simulink model "Square"  (R2012b)
settings: Solver=ode1  StartTime=0.0  StopTime=inf  FixedStep=0.002  RelTol=1e-3
undefined symbols (not defined in the file): qc_get_step_size
libraries: simulink x33, simulink_extras x8, quarc_library x2
settings Model: ExtModeTrigDuration=5000  Creator=user  LastModifiedBy=user
settings SolverCC: PositivePriorityOrder=on
settings RTWCC: SystemTargetFile=quarc_win64.tlc  TemplateMakefile=quarc_default_tmf  Description=QUARC Win64 Target  ProcessScript=quarc_win64_make_rtw_hook
settings STFCustomTargetCC: TargetPreCompLibLocation=C:\PROGRA~3\QUARC\lib\2012b\win64\release  CodeReplacementLibrary=ANSI_C  GeneratePreprocessorConditionals=Disable all  CombineOutputUpdateFcns=on  GRTInterface=off  SystemTargetFile=quarc_win64.tlc
settings GRTTargetCC: TargetPreCompLibLocation=C:\PROGRA~3\QUARC\lib\2012b\win64\release  ParMdlRefBuildCompliant=off  CompOptLevelCompliant=off  ConcurrentExecutionCompliant=off  MatFileLogging=off  ExtMode=on  ExtModeMexFile=quarc_comm

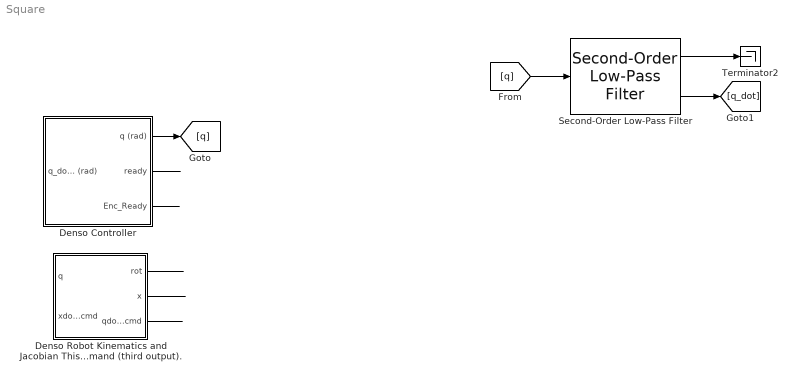
== system Square ==
  Denso Controller : Subsystem
  Denso Robot Kinematics and Jacobian This block takes the joint values of the robot as the first input and calculates the rotational matrix and position of the robot end-effector in the global frame (first two outputs). It also takes the speed command in the global frame (second input) and converts it to joint speed command (third output). : Subsystem
  Second-Order Low-Pass Filter : quarc_library/Continuous/Second-Order Low-Pass Filter  params_source=Internal (dialog parameters)  input_width=1  input_zeta=1  input_init=0
  Terminator2 : Terminator
  wires:
  [q] -> Second-Order Low-Pass Filter/1
  Denso Controller/1(q (rad)) -> [q]
  Second-Order Low-Pass Filter/1 -> Terminator2/1
  Second-Order Low-Pass Filter/2 -> [q_dot]
  Denso Robot Kinematics and Jacobian This block takes the joint values of the robot as the first input and calculates the rotational matrix and position of the robot end-effector in the global frame (first two outputs). It also takes the speed command in the global frame (second input) and converts it to joint speed command (third output)./1(rot) -> ?
  Denso Robot Kinematics and Jacobian This block takes the joint values of the robot as the first input and calculates the rotational matrix and position of the robot end-effector in the global frame (first two outputs). It also takes the speed command in the global frame (second input) and converts it to joint speed command (third output)./2(x) -> ?
  Denso Controller/2(ready) -> ?
  Denso Controller/3(Enc_Ready) -> ?
  ? -> Denso Controller/1(q_dot_cmd (rad))
  Denso Robot Kinematics and Jacobian This block takes the joint values of the robot as the first input and calculates the rotational matrix and position of the robot end-effector in the global frame (first two outputs). It also takes the speed command in the global frame (second input) and converts it to joint speed command (third output)./3(qdot_cmd) -> ?

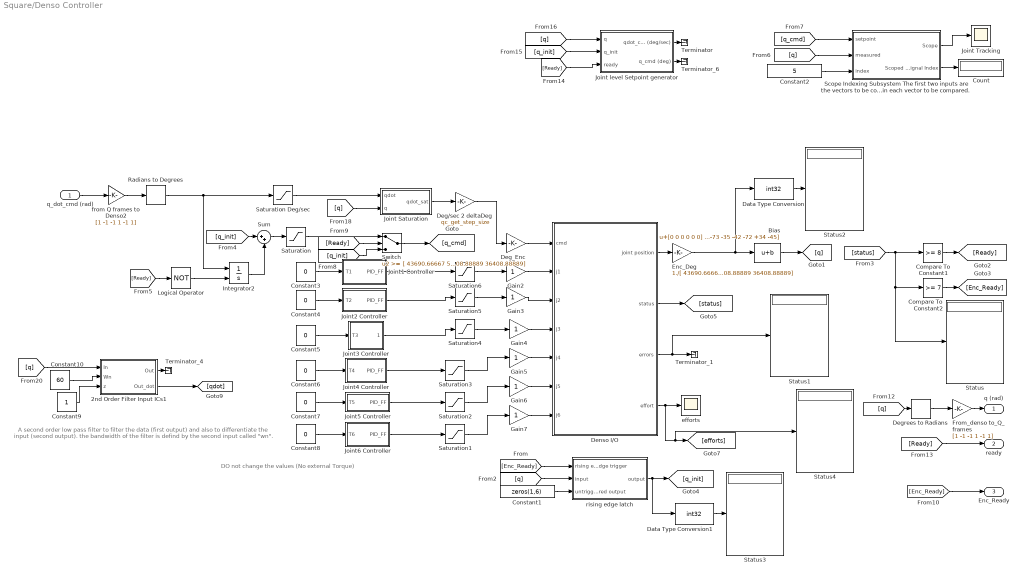
== system Square/Denso Controller ==
  note: DO not change the values (No external Torque)
  note: A second order low pass filter to filter the data (first output) and also to differentiate
      |  the input (second output). the bandwidth of the filter is defind by the second input called "wn".
  q_dot_cmd (rad) : Inport
  2nd Order Filter Input ICs1 : Subsystem
  Bias : Bias  Bias=[0 0 0 0 0 0] %0*[-146 -102 -137+90 -155 85+90 -370]%[-73 -35 -42 -72 +34 -45]
  Compare To Constant1 : simulink/Logic and Bit Operations/Compare To Constant  relop=>=  const=8  OutDataTypeStr=uint8  ZeroCross=off
  Compare To Constant2 : simulink/Logic and Bit Operations/Compare To Constant  relop=>=  const=7  OutDataTypeStr=uint8  ZeroCross=off
  Constant1 : Constant  Value=zeros(1,6)
  Constant10 : Constant  Value=60
  Constant2 : Constant  Value=5
  Constant{3..8} (6 alike) : Constant  Value=0
  Constant9 : Constant
  Count : Display
      settings: Decimation=100
  Data Type Conversion : DataTypeConversion  OutDataTypeStr=int32
  Data Type Conversion1 : DataTypeConversion  OutDataTypeStr=int32
  Deg/sec 2 deltaDeg : Gain  Gain=qc_get_step_size
  Deg_Enc : Gain  Gain=[ 43690.66667 58254.22222 43690.66667 36408.88889 36408.88889 36408.88889]
  Degrees to Radians : simulink_extras/Transformations/Degrees to Radians
  Denso I/O : Subsystem
  Enc_Deg : Gain  Gain=1./[ 43690.66667 58254.22222 43690.66667 36408.88889 36408.88889 36408.88889]
  From_denso to_Q_frames : Gain  Gain=[1 -1 -1 1 -1 1]
  Gain{2..7} (6 alike) : Gain
  Integrator2 : Integrator  ExternalReset=level
  Joint Saturation : Subsystem
  Joint Tracking : Scope
      settings: TimeRange=2  YMin=93  YMax=100.5
  Joint level Setpoint generator : Subsystem
  Joint1 Controller : Subsystem
  Joint2 Controller : Subsystem
  Joint3 Controller : Subsystem
  Joint4 Controller : Subsystem
  Joint5 Controller : Subsystem
  Joint6 Controller : Subsystem
  Logical Operator : Logic  Operator=NOT  AllPortsSameDT=off  OutDataTypeStr=boolean
  Radians to Degrees : simulink_extras/Transformations/Radians to Degrees
  Saturation : Saturate  UpperLimit=[160 65 162 162 100 365]  LowerLimit=-[160 122 20 162 100 365]
  Saturation Deg/sec : Saturate  UpperLimit="1e3*[1.1444    0.8583    1.1444    1.3733    1.3733    1.3733]"  LowerLimit="-1e3*[1.1444    0.8583    1.1444    1.3733    1.3733    1.3733]"
  Saturation{1..6} (6 alike) : Saturate  UpperLimit=3.7  LowerLimit=-3.7
  Scope Indexing Subsystem The first two inputs are the vectors to be compared. The third input is an index to define the elements in each vector to be compared. : Subsystem
  Status{,1..4} (5 alike) : Display
      settings: Decimation=100
  Sum : Sum  Inputs=|++
  Switch : Switch  Threshold=1
  Terminator : Terminator
  Terminator_1 : Terminator
  Terminator_4 : Terminator
  Terminator_6 : Terminator
  efforts : Scope
      settings: TimeRange=2  YMin=-4.5  YMax=0.5  SaveName=ScopeData3
  from Q frames to Denso2 : Gain  Gain=[1 -1 -1 1 -1 1]
  rising edge latch : Subsystem
  q (rad) : Outport
  ready : Outport  Port=2
  Enc_Ready : Outport  Port=3
  wires:
  Denso I/O/1(joint position) -> Enc_Deg/1
  Enc_Deg/1 -> Data Type Conversion/1, Bias/1
  Gain2/1 -> Denso I/O/2(j1)
  Gain3/1 -> Denso I/O/3(j2)
  Gain4/1 -> Denso I/O/4(j3)
  Gain5/1 -> Denso I/O/5(j4)
  Gain6/1 -> Denso I/O/6(j5)
  Gain7/1 -> Denso I/O/7(j6)
  Joint2 Controller/1(PID_FF) -> Saturation5/1
  Joint3 Controller/1(PID_FF) -> Saturation4/1
  Joint1 Controller/1(PID_FF) -> Saturation6/1
  [Enc_Ready] -> rising edge latch/1(rising edge trigger)
  Compare To Constant1/1 -> [Ready]
  [q] -> rising edge latch/2(input)
  rising edge latch/1(output) -> [q_init], Data Type Conversion1/1
  Constant1/1 -> rising edge latch/3(untriggered output)
  Denso I/O/4(effort) -> efforts/1, [efforts], Status4/1
  Scope Indexing Subsystem The first two inputs are the vectors to be compared. The third input is an index to define the elements in each vector to be compared./2(Scoped Signal Index) -> Count/1
  Constant2/1 -> Scope Indexing Subsystem The first two inputs are the vectors to be compared. The third input is an index to define the elements in each vector to be compared./3(index)
  Compare To Constant2/1 -> [Enc_Ready]
  Denso I/O/2(status) -> [status]
  [status] -> Compare To Constant1/1, Compare To Constant2/1, Status/1
  [q_cmd] -> Scope Indexing Subsystem The first two inputs are the vectors to be compared. The third input is an index to define the elements in each vector to be compared./1(setpoint)
  [q] -> Scope Indexing Subsystem The first two inputs are the vectors to be compared. The third input is an index to define the elements in each vector to be compared./2(measured)
  [Ready] -> Logical Operator/1
  Logical Operator/1 -> Integrator2/2
  q_dot_cmd (rad)/1 -> from Q frames to Denso2/1
  [q] -> Degrees to Radians/1
  [Ready] -> ready/1
  [Enc_Ready] -> Enc_Ready/1
  Denso I/O/3(errors) -> Terminator_1/1, Status1/1
  Degrees to Radians/1 -> From_denso to_Q_frames/1
  Deg/sec 2 deltaDeg/1 -> Deg_Enc/1
  From_denso to_Q_frames/1 -> q (rad)/1
  [q] -> 2nd Order Filter Input ICs1/1(In)
  Constant9/1 -> 2nd Order Filter Input ICs1/3(z)
  Constant10/1 -> 2nd Order Filter Input ICs1/2(Wn)
  2nd Order Filter Input ICs1/2(Out_dot) -> [qdot]
  Joint4 Controller/1(PID_FF) -> Saturation3/1
  Joint5 Controller/1(PID_FF) -> Saturation2/1
  Joint6 Controller/1(PID_FF) -> Saturation1/1
  2nd Order Filter Input ICs1/1(Out) -> Terminator_4/1
  [q] -> Joint level Setpoint generator/1(q)
  [q_init] -> Joint level Setpoint generator/2(q_init)
  [Ready] -> Joint level Setpoint generator/3(ready)
  Joint level Setpoint generator/2(q_cmd (deg)) -> Terminator_6/1
  Saturation Deg/sec/1 -> Joint Saturation/1(qdot)
  [q] -> Joint Saturation/2(q)
  from Q frames to Denso2/1 -> Radians to Degrees/1
  Scope Indexing Subsystem The first two inputs are the vectors to be compared. The third input is an index to define the elements in each vector to be compared./1(Scope) -> Joint Tracking/1
  Data Type Conversion/1 -> Status2/1
  Data Type Conversion1/1 -> Status3/1
  Joint Saturation/1(qdot_sat) -> Deg/sec 2 deltaDeg/1
  Bias/1 -> [q]
  [Ready] -> Switch/2
  Sum/1 -> Saturation/1
  Switch/1 -> [q_cmd]
  [q_init] -> Switch/3
  [q_init] -> Sum/1
  Integrator2/1 -> Sum/2
  Saturation/1 -> Switch/1
  Radians to Degrees/1 -> Integrator2/1, Saturation Deg/sec/1
  Deg_Enc/1 -> Denso I/O/1(cmd)
  Constant3/1 -> Joint1 Controller/1(T1)
  Constant4/1 -> Joint2 Controller/1(T2)
  Constant5/1 -> Joint3 Controller/1(T3)
  Constant6/1 -> Joint4 Controller/1(T4)
  Constant7/1 -> Joint5 Controller/1(T5)
  Saturation1/1 -> Gain7/1
  Saturation2/1 -> Gain6/1
  Saturation3/1 -> Gain5/1
  Saturation4/1 -> Gain4/1
  Saturation5/1 -> Gain3/1
  Saturation6/1 -> Gain2/1
  Constant8/1 -> Joint6 Controller/1(T6)
  Joint level Setpoint generator/1(qdot_cmd (deg/sec)) -> Terminator/1

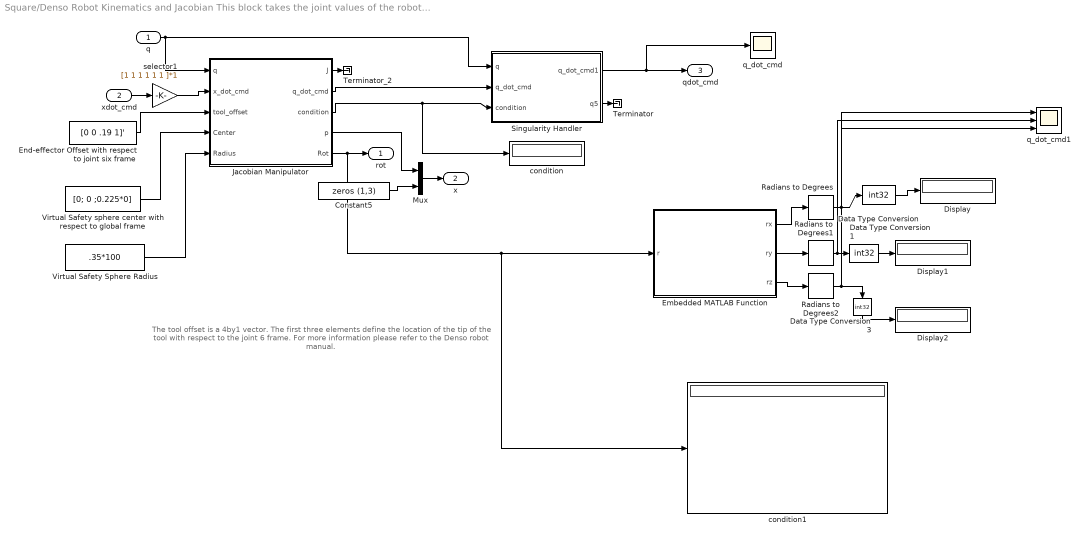
== system Square/Denso Robot Kinematics and Jacobian This block takes the joint values of the robot as the first input and calculates the rotational matrix and position of the robot end-effector in the global frame (first two outputs). It also takes the speed command in the global frame (second input) and converts it to joint speed command (third output). ==
  note: The tool offset is a 4by1 vector. The first three elements define
      | the location of the tip of the tool with respect to the joint 6 frame.
      | For more information please refer to the Denso robot manual.
  q : Inport
  xdot_cmd : Inport  Port=2
  Constant5 : Constant  Value=zeros (1,3)
  Data Type Conversion : DataTypeConversion  OutDataTypeStr=int32
  Data Type Conversion1 : DataTypeConversion  OutDataTypeStr=int32
  Data Type Conversion3 : DataTypeConversion  OutDataTypeStr=int32
  Display : Display
      settings: Decimation=100
  Display1 : Display
      settings: Decimation=100
  Display2 : Display
      settings: Decimation=100
  Embedded MATLAB Function : MATLAB Function  TreatAsAtomicUnit=on
  End-effector Offset with respect to joint six frame : Constant  Value=[0 0 .19 1]'
  Jacobian Manipulator : Subsystem
  Mux : Mux  Inputs=2
  Radians to Degrees : simulink_extras/Transformations/Radians to Degrees
  Radians to Degrees1 : simulink_extras/Transformations/Radians to Degrees
  Radians to Degrees2 : simulink_extras/Transformations/Radians to Degrees
  Singularity Handler : Subsystem
  Terminator : Terminator
  Terminator_2 : Terminator
  Virtual Safety Sphere Radius : Constant  Value=.35*100
  Virtual Safety sphere center with respect to global frame : Constant  Value=[0; 0 ;0.225*0]
  condition : Display
      settings: Decimation=100
  condition1 : Display
      settings: Decimation=100
  q_dot_cmd : Scope
      settings: TimeRange=2  YMin=-2.75e-005  YMax=2.75e-005  SaveName=ScopeData19
  q_dot_cmd1 : Scope  NumInputPorts=3
      settings: TimeRange=2  YMin=-2.75e-005~-5~-5  YMax=2.75e-005~5~5  SaveName=ScopeData5
  selector1 : Gain  Gain=[1 1 1 1 1 1 ]*1
  rot : Outport
  x : Outport  Port=2
  qdot_cmd : Outport  Port=3
  wires:
  Jacobian Manipulator/1(J) -> Terminator_2/1
  Constant5/1 -> Mux/2
  selector1/1 -> Jacobian Manipulator/2(x_dot_cmd)
  Jacobian Manipulator/3(condition) -> Singularity Handler/3(condition), condition/1
  Jacobian Manipulator/4(p) -> Mux/1
  Singularity Handler/1(q_dot_cmd1) -> q_dot_cmd/1, qdot_cmd/1
  End-effector Offset with respect to joint six frame/1 -> Jacobian Manipulator/3(tool_offset)
  Jacobian Manipulator/2(q_dot_cmd) -> Singularity Handler/2(q_dot_cmd)
  q/1 -> Jacobian Manipulator/1(q), Singularity Handler/1(q)
  xdot_cmd/1 -> selector1/1
  Jacobian Manipulator/5(Rot) -> rot/1, Embedded MATLAB Function/1(r), condition1/1
  Mux/1 -> x/1
  Virtual Safety sphere center with respect to global frame/1 -> Jacobian Manipulator/4(Center)
  Virtual Safety Sphere Radius/1 -> Jacobian Manipulator/5(Radius)
  Embedded MATLAB Function/1(rx) -> Radians to Degrees/1
  Embedded MATLAB Function/2(ry) -> Radians to Degrees1/1
  Embedded MATLAB Function/3(rz) -> Radians to Degrees2/1
  Radians to Degrees/1 -> Data Type Conversion/1, q_dot_cmd1/1
  Radians to Degrees1/1 -> Data Type Conversion1/1, q_dot_cmd1/2
  Radians to Degrees2/1 -> Data Type Conversion3/1, q_dot_cmd1/3
  Data Type Conversion/1 -> Display/1
  Data Type Conversion1/1 -> Display1/1
  Data Type Conversion3/1 -> Display2/1
  Singularity Handler/2(q5) -> Terminator/1

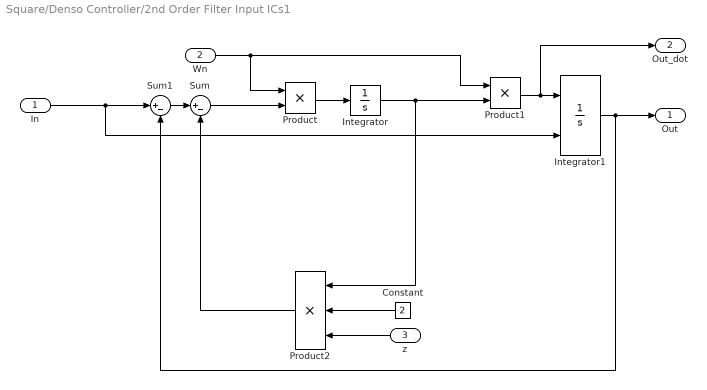
== system Square/Denso Controller/2nd Order Filter Input ICs1 ==
  In : Inport
  Wn : Inport  Port=2
  z : Inport  Port=3
  Constant : Constant  Value=2
  Integrator : Integrator
  Integrator1 : Integrator  InitialConditionSource=external
  Product : Product  RndMeth=Zero
  Product1 : Product  RndMeth=Zero
  Product2 : Product  Inputs=3  RndMeth=Zero
  Sum : Sum  Inputs=|+-
  Sum1 : Sum  Inputs=|+-
  Out : Outport
  Out_dot : Outport  Port=2
  wires:
  Constant/1 -> Product2/2
  z/1 -> Product2/3
  Product2/1 -> Sum/2
  In/1 -> Integrator1/2, Sum1/1
  Sum1/1 -> Sum/1
  Integrator1/1 -> Out/1, Sum1/2
  Integrator/1 -> Product2/1, Product1/2
  Product1/1 -> Out_dot/1, Integrator1/1
  Wn/1 -> Product1/1, Product/1
  Sum/1 -> Product/2
  Product/1 -> Integrator/1

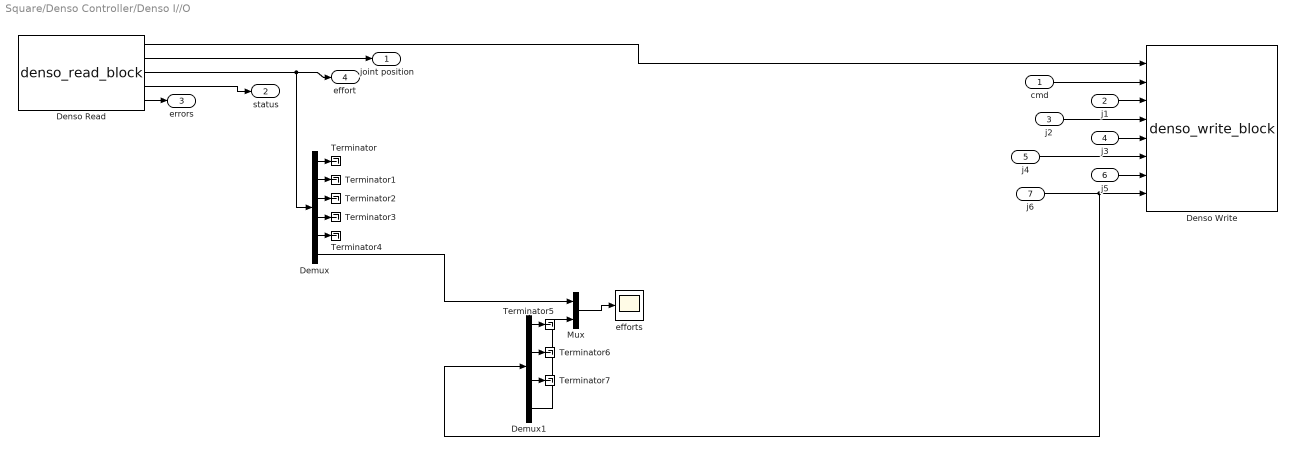
== system Square/Denso Controller/Denso I//O ==
  cmd : Inport
  j1 : Inport  Port=2
  j2 : Inport  Port=3
  j3 : Inport  Port=4
  j4 : Inport  Port=5
  j5 : Inport  Port=6
  j6 : Inport  Port=7
  Demux : Demux  Outputs=6
  Demux1 : Demux
  Denso Read : S-Function  FunctionName=denso_read_block  Parameters=uri  EnableBusSupport=off  mask(Denso Read){uri=udp://192.168.0.1:1000}
      mask help: Initializes a connection to the Denso robot controller and reads the robot joint positions and state.
      mask init:
      | commands = { ...
      |     'port_label(''output'', 1, ''denso'');', ...
      |     'port_label(''output'', 2, ''position'');', ...
      |     'port_label(''output'', 3, ''effort'');', ...
      |     'port_label(''output'', 4, ''status'');' ...
      |     'port_label(''output'', 5, ''errors'');' ...
      | };
      | 
      | qc_set_display('Denso Read', commands);
      mask Display:
      | patch([0.98591 0.98591 0.62618 0.59072 0.56147   0.536   0.536  0.5441 0.56912 0.59207 0.60881 0.62276 0.63527 0.64364  0.6485  0.6485 0.64706 0.64499 0.63662 0.62411 0.61232 0.59837 0.58307 0.56147   0.536   0.536  0.5441  0.5747 0.60953 0.63662 0.67001  0.7034 0.72851 0.75425 0.77927 0.80294 0.82454 0.84119 0.85865 0.87395 0.88574 0.89339  0.8969 0.89969 0.89969 0.89267  0.8816 0.87044 0.85649  0.8384 0.81824 0.80294 0.78764 0.77513 0.76676 0.75776 0.76397 0.77513 0.79178 0.80987 0.82796 0.84326 0.86207 0.98528],[0.18689 0.05522 0.05522 0.05171 0.05171    0.05 0.18338 0.18338 0.19148 0.20435 0.22298 0.24863 0.28589 0.33125 0.38138 0.55139 0.59801 0.63761 0.68189 0.72149 0.74939 0.76694 0.77855 0.79367 0.79952 0.92768 0.92768 0.92768 0.92417 0.92066 0.91364  0.9032 0.89384 0.88106 0.86594 0.85073 0.82634 0.80537 0.77855 0.74363 0.70403 0.65858 0.61079 0.59099 0.41513 0.37202 0.31847 0.29048 0.25556 0.23342  0.2102 0.19382 0.18221 0.17285 0.16943 0.16124  0.1589 0.16241 0.16709 0.17168  0.1787 0.18221 0.18689 0.18689],[0.9,0.90,0.91])
      | patch([0.536 0.52601 0.46823 0.44528 0.41603 0.39101 0.35555 0.33116 0.31451 0.29291  0.2804 0.26717 0.25322 0.23999 0.22406 0.20732 0.19337 0.17528 0.15935 0.14396 0.13217 0.11759 0.10922 0.10085 0.09671 0.09392 0.09041 0.08906 0.08906 0.09464  0.0995 0.10778 0.11894 0.13145 0.14675 0.16349 0.17672 0.19409 0.20732 0.22406 0.23999 0.26159 0.27833 0.29849 0.31793 0.33602 0.35411 0.37085 0.39245 0.41603   0.536   0.536 0.53159 0.46409   0.446 0.42026 0.39587 0.37571 0.36113 0.34925 0.34088 0.33809 0.33809 0.34088 0.34583 0.35627 0.36392 0.38129 0.39587 0.41117 0.42719 0.44672  0.4676 0.48353 0.48353 0.52394   0.536],[0.05 0.04829 0.04712 0.04712 0.04829 0.05063 0.05405 0.05873 0.06107 0.06692 0.07043 0.07619 0.08087 0.08672 0.09482 0.10652 0.11696 0.13325  0.1508 0.17168 0.19499 0.22415 0.25439 0.28472 0.31379 0.35456 0.38489 0.41513 0.58055 0.63878 0.68774 0.72149 0.75641 0.78089 0.80537 0.82859 0.84029 0.85658 0.86594 0.87404  0.8834 0.89267 0.90086 0.90788 0.91247 0.91832 0.92066   0.923 0.92651 0.92768 0.92768 0.79952 0.79952 0.79952 0.79718 0.78899 0.77153 0.75056 0.72149 0.68072 0.62249  0.5549 0.41396 0.37085 0.33242 0.28121 0.25205 0.22181 0.20552 0.19499 0.18572 0.18221 0.17753 0.17636 0.17753  0.1787  0.1787],[0.9,0.90,0.91])
      | disp('Denso Read');
      | port_label('output', 1, 'denso');
      | port_label('output', 2, 'position');
      | port_label('output', 3, 'effort');
      | port_label('output', 4, 'status');
      | port_label('output', 5, 'errors');
  Denso Write : S-Function  FunctionName=denso_write_block  Parameters=velocity_mode  EnableBusSupport=off  mask(Denso Write){velocity_mode=on}
      mask prompts: velocity_mode "Velocity mode"
      mask help: Sends joint commands and controller gains to the Denso robot.
      mask init:
      | commands = { ...
      |     'port_label(''input'', 1, ''denso'');', ...
      |     'port_label(''input'', 2, ''command'');', ...
      |     'port_label(''input'', 3, ''J1 gains'');', ...
      |     'port_label(''input'', 4, ''J2 gains'');' ...
      |     'port_label(''input'', 5, ''J3 gains'');' ...
      |     'port_label(''input'', 6, ''J4 gains'');' ...
      |     'port_label(''input'', 7, ''J5 gains'');' ...
      |     'port_label(''input'', 8, ''J6 gains'');' ...
      | };
      | 
      | qc_set_display('Denso Write', commands);
      mask Display:
      | patch([0.98591 0.98591 0.62618 0.59072 0.56147   0.536   0.536  0.5441 0.56912 0.59207 0.60881 0.62276 0.63527 0.64364  0.6485  0.6485 0.64706 0.64499 0.63662 0.62411 0.61232 0.59837 0.58307 0.56147   0.536   0.536  0.5441  0.5747 0.60953 0.63662 0.67001  0.7034 0.72851 0.75425 0.77927 0.80294 0.82454 0.84119 0.85865 0.87395 0.88574 0.89339  0.8969 0.89969 0.89969 0.89267  0.8816 0.87044 0.85649  0.8384 0.81824 0.80294 0.78764 0.77513 0.76676 0.75776 0.76397 0.77513 0.79178 0.80987 0.82796 0.84326 0.86207 0.98528],[0.18689 0.05522 0.05522 0.05171 0.05171    0.05 0.18338 0.18338 0.19148 0.20435 0.22298 0.24863 0.28589 0.33125 0.38138 0.55139 0.59801 0.63761 0.68189 0.72149 0.74939 0.76694 0.77855 0.79367 0.79952 0.92768 0.92768 0.92768 0.92417 0.92066 0.91364  0.9032 0.89384 0.88106 0.86594 0.85073 0.82634 0.80537 0.77855 0.74363 0.70403 0.65858 0.61079 0.59099 0.41513 0.37202 0.31847 0.29048 0.25556 0.23342  0.2102 0.19382 0.18221 0.17285 0.16943 0.16124  0.1589 0.16241 0.16709 0.17168  0.1787 0.18221 0.18689 0.18689],[0.9,0.90,0.91])
      | patch([0.536 0.52601 0.46823 0.44528 0.41603 0.39101 0.35555 0.33116 0.31451 0.29291  0.2804 0.26717 0.25322 0.23999 0.22406 0.20732 0.19337 0.17528 0.15935 0.14396 0.13217 0.11759 0.10922 0.10085 0.09671 0.09392 0.09041 0.08906 0.08906 0.09464  0.0995 0.10778 0.11894 0.13145 0.14675 0.16349 0.17672 0.19409 0.20732 0.22406 0.23999 0.26159 0.27833 0.29849 0.31793 0.33602 0.35411 0.37085 0.39245 0.41603   0.536   0.536 0.53159 0.46409   0.446 0.42026 0.39587 0.37571 0.36113 0.34925 0.34088 0.33809 0.33809 0.34088 0.34583 0.35627 0.36392 0.38129 0.39587 0.41117 0.42719 0.44672  0.4676 0.48353 0.48353 0.52394   0.536],[0.05 0.04829 0.04712 0.04712 0.04829 0.05063 0.05405 0.05873 0.06107 0.06692 0.07043 0.07619 0.08087 0.08672 0.09482 0.10652 0.11696 0.13325  0.1508 0.17168 0.19499 0.22415 0.25439 0.28472 0.31379 0.35456 0.38489 0.41513 0.58055 0.63878 0.68774 0.72149 0.75641 0.78089 0.80537 0.82859 0.84029 0.85658 0.86594 0.87404  0.8834 0.89267 0.90086 0.90788 0.91247 0.91832 0.92066   0.923 0.92651 0.92768 0.92768 0.79952 0.79952 0.79952 0.79718 0.78899 0.77153 0.75056 0.72149 0.68072 0.62249  0.5549 0.41396 0.37085 0.33242 0.28121 0.25205 0.22181 0.20552 0.19499 0.18572 0.18221 0.17753 0.17636 0.17753  0.1787  0.1787],[0.9,0.90,0.91])
      | disp('Denso Write');
      | port_label('input', 1, 'denso');
      | port_label('input', 2, 'command');
      | port_label('input', 3, 'J1 gains');
      | port_label('input', 4, 'J2 gains');
      | port_label('input', 5, 'J3 gains');
      | port_label('input', 6, 'J4 gains');
      | port_label('input', 7, 'J5 gains');
      | port_label('input', 8, 'J6 gains');
  Mux : Mux  Inputs=2
  Terminator{,1..7} (8 alike) : Terminator
  efforts : Scope
      settings: TimeRange=2  YMin=-4.5  YMax=0.5  SaveName=compare
  joint position : Outport
  status : Outport  Port=2
  errors : Outport  Port=3
  effort : Outport  Port=4
  wires:
  j6/1 -> Demux1/1, Denso Write/8
  j5/1 -> Denso Write/7
  j4/1 -> Denso Write/6
  j3/1 -> Denso Write/5
  j2/1 -> Denso Write/4
  j1/1 -> Denso Write/3
  Denso Read/5 -> errors/1
  Denso Read/4 -> status/1
  Denso Read/3 -> Demux/1, effort/1
  Denso Read/2 -> joint position/1
  Denso Read/1 -> Denso Write/1
  cmd/1 -> Denso Write/2
  Demux/6 -> Mux/1
  Mux/1 -> efforts/1
  Demux1/4 -> Mux/2
  Demux/1 -> Terminator/1
  Demux/2 -> Terminator1/1
  Demux/3 -> Terminator2/1
  Demux/4 -> Terminator3/1
  Demux/5 -> Terminator4/1
  Demux1/1 -> Terminator5/1
  Demux1/2 -> Terminator6/1
  Demux1/3 -> Terminator7/1

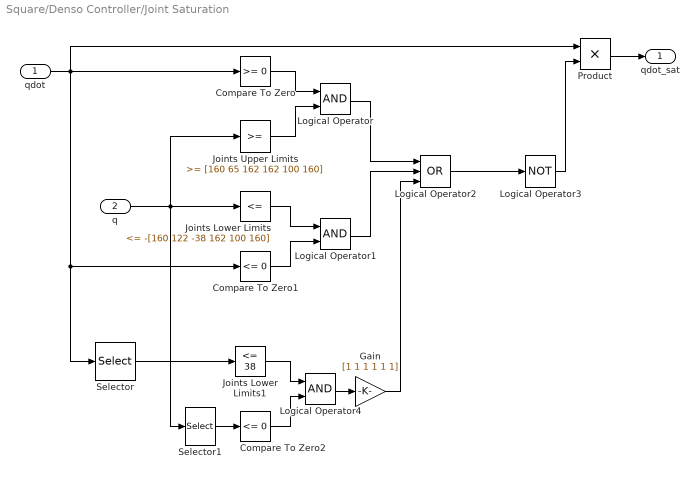
== system Square/Denso Controller/Joint Saturation ==
  qdot : Inport
  q : Inport  Port=2
  Compare To Zero : simulink/Logic and Bit Operations/Compare To Zero  relop=>=  OutDataTypeStr=uint8  ZeroCross=off
  Compare To Zero1 : simulink/Logic and Bit Operations/Compare To Zero  relop=<=  OutDataTypeStr=uint8  ZeroCross=off
  Compare To Zero2 : simulink/Logic and Bit Operations/Compare To Zero  relop=<=  OutDataTypeStr=uint8  ZeroCross=off
  Gain : Gain  Gain=[1 1 1 1 1 1]
  Joints Lower Limits : simulink/Logic and Bit Operations/Compare To Constant  relop=<=  const=-[160 122 -38 162 100 160]  OutDataTypeStr=uint8  ZeroCross=off
  Joints Lower Limits1 : simulink/Logic and Bit Operations/Compare To Constant  relop=<=  const=38  OutDataTypeStr=uint8  ZeroCross=off
  Joints Upper Limits : simulink/Logic and Bit Operations/Compare To Constant  relop=>=  const=[160 65 162 162 100 160]  OutDataTypeStr=uint8  ZeroCross=off
  Logical Operator : Logic  AllPortsSameDT=off  OutDataTypeStr=boolean
  Logical Operator1 : Logic  AllPortsSameDT=off  OutDataTypeStr=boolean
  Logical Operator2 : Logic  Operator=OR  Inputs=3  AllPortsSameDT=off  OutDataTypeStr=boolean
  Logical Operator3 : Logic  Operator=NOT  AllPortsSameDT=off  OutDataTypeStr=boolean
  Logical Operator4 : Logic  AllPortsSameDT=off  OutDataTypeStr=boolean
  Product : Product  RndMeth=Zero
  Selector : Selector  InputPortWidth=6  IndexOptions=Index vector (dialog)  Indices=3  OutputSizes=1
  Selector1 : Selector  InputPortWidth=6  IndexOptions=Index vector (dialog)  Indices=3  OutputSizes=1
  qdot_sat : Outport
  wires:
  q/1 -> Joints Lower Limits/1, Joints Upper Limits/1, Selector1/1
  Logical Operator2/1 -> Logical Operator3/1
  Compare To Zero/1 -> Logical Operator/1
  Joints Upper Limits/1 -> Logical Operator/2
  Joints Lower Limits/1 -> Logical Operator1/1
  Compare To Zero1/1 -> Logical Operator1/2
  Logical Operator/1 -> Logical Operator2/1
  Logical Operator1/1 -> Logical Operator2/2
  qdot/1 -> Compare To Zero/1, Product/1, Compare To Zero1/1, Selector/1
  Logical Operator3/1 -> Product/2
  Product/1 -> qdot_sat/1
  Joints Lower Limits1/1 -> Logical Operator4/1
  Compare To Zero2/1 -> Logical Operator4/2
  Selector/1 -> Joints Lower Limits1/1
  Selector1/1 -> Compare To Zero2/1
  Logical Operator4/1 -> Gain/1
  Gain/1 -> Logical Operator2/3

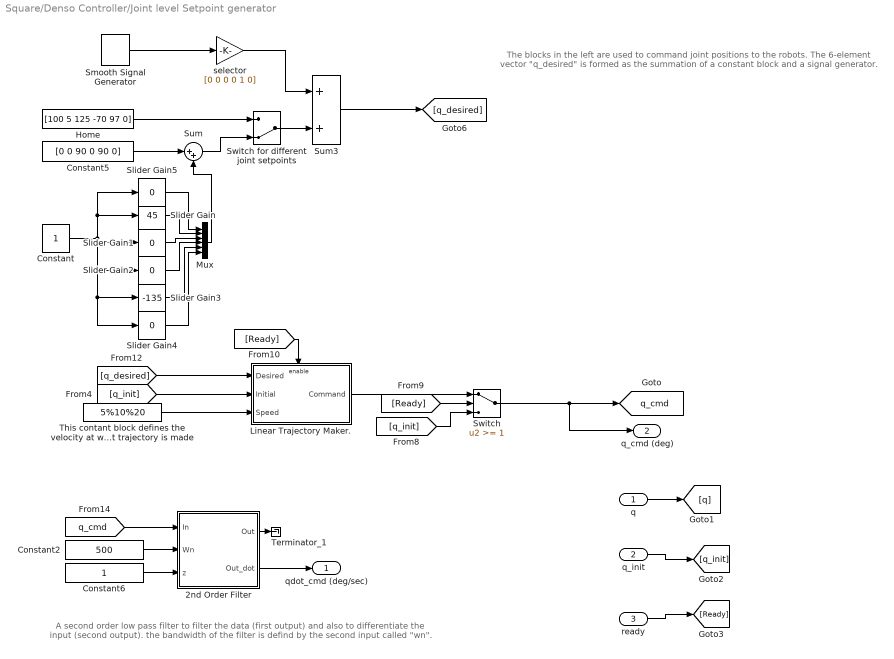
== system Square/Denso Controller/Joint level Setpoint generator ==
  note: A second order low pass filter to filter the data (first output) and also to differentiate
      |  the input (second output). the bandwidth of the filter is defind by the second input called "wn".
  note: The blocks in the left are used to command joint positions to the robots. The 6-element vector "q_desired" is formed as
      | the summation of a constant block and a signal generator.
  q : Inport
  q_init : Inport  Port=2
  ready : Inport  Port=3
  2nd Order Filter : Subsystem
  Constant : Constant
  Constant2 : Constant  Value=500
  Constant5 : Constant  Value=[0 0 90 0 90 0]
  Constant6 : Constant
  Home : Constant  Value=[100 5 125 -70 97 0]
  Linear Trajectory Maker. : Subsystem  TreatAsAtomicUnit=on
  Mux : Mux  Inputs=6
  Slider Gain : simulink/Math Operations/Slider Gain  low=-10  gain=45  high=45
  Slider Gain1 : simulink/Math Operations/Slider Gain  low=-60  gain=0  high=10
  Slider Gain2 : simulink/Math Operations/Slider Gain  low=-10  gain=0  high=10
  Slider Gain3 : simulink/Math Operations/Slider Gain  low=-180  gain=-135  high=10
  Slider Gain4 : simulink/Math Operations/Slider Gain  low=-10  gain=0  high=10
  Slider Gain5 : simulink/Math Operations/Slider Gain  low=-10  gain=0  high=10
  Smooth Signal Generator : quarc_library/Sources/Signals/Smooth Signal Generator  signal_type=Sine  source=Internal (dialog parameters)  amplitude=0  frequency=.2  initial_phase=0  sample_time=qc_get_step_size  output_cos=off
  Sum : Sum  Inputs=|++
  Sum3 : Sum
  Switch : Switch  Threshold=1
  Switch for different joint setpoints : ManualSwitch  CurrentSetting=0
  Terminator_1 : Terminator
  This contant block defines the velocity at which the desired joint trajectory is made : Constant  Value=5%10%20
  selector : Gain  Gain=[0 0 0 0 1 0]
  qdot_cmd (deg/sec) : Outport
  q_cmd (deg) : Outport  Port=2
  tag scope: q_cmd=global
  wires:
  [Ready] -> Switch/2
  Linear Trajectory Maker./1(Command) -> Switch/1
  [Ready] -> Linear Trajectory Maker./Enable
  This contant block defines the velocity at which the desired joint trajectory is made/1 -> Linear Trajectory Maker./3(Speed)
  [q_init] -> Switch/3
  [q_init] -> Linear Trajectory Maker./2(Initial)
  selector/1 -> Sum3/1
  Sum3/1 -> [q_desired]
  Home/1 -> Switch for different joint setpoints/1
  [q_desired] -> Linear Trajectory Maker./1(Desired)
  Switch for different joint setpoints/1 -> Sum3/2
  Constant2/1 -> 2nd Order Filter/2(Wn)
  Constant6/1 -> 2nd Order Filter/3(z)
  Switch/1 -> [q_cmd], q_cmd (deg)/1
  2nd Order Filter/2(Out_dot) -> qdot_cmd (deg/sec)/1
  q/1 -> [q]
  q_init/1 -> [q_init]
  ready/1 -> [Ready]
  2nd Order Filter/1(Out) -> Terminator_1/1
  [q_cmd] -> 2nd Order Filter/1(In)
  Smooth Signal Generator/1 -> selector/1
  Constant5/1 -> Sum/1
  Constant/1 -> Slider Gain5/1, Slider Gain/1, Slider Gain1/1, Slider Gain2/1, Slider Gain3/1, Slider Gain4/1
  Slider Gain5/1 -> Mux/1
  Slider Gain/1 -> Mux/2
  Slider Gain1/1 -> Mux/3
  Slider Gain2/1 -> Mux/4
  Slider Gain3/1 -> Mux/5
  Slider Gain4/1 -> Mux/6
  Mux/1 -> Sum/2
  Sum/1 -> Switch for different joint setpoints/2

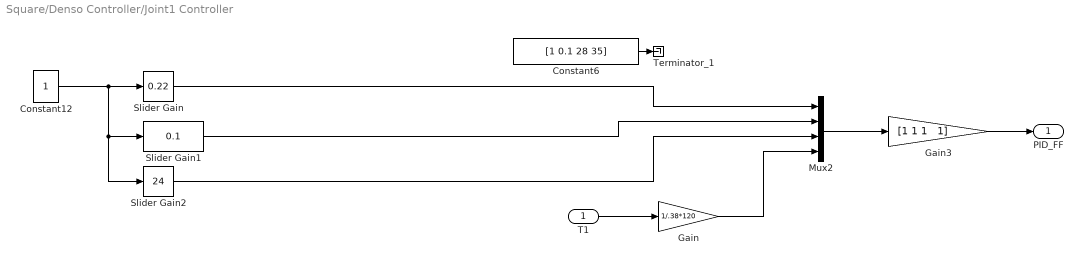
== system Square/Denso Controller/Joint1 Controller ==
  T1 : Inport
  Constant12 : Constant
  Constant6 : Constant  Value=[1 0.1 28 35]
  Gain : Gain  Gain=1/.38*120
  Gain3 : Gain  Gain="[1 1 1   1]"
  Mux2 : Mux
  Slider Gain : simulink/Math Operations/Slider Gain  low=0  gain=0.22  high=1
  Slider Gain1 : simulink/Math Operations/Slider Gain  low=0  gain=0.1  high=24
  Slider Gain2 : simulink/Math Operations/Slider Gain  low=0  gain=24  high=100
  Terminator_1 : Terminator
  PID_FF : Outport
  wires:
  Mux2/1 -> Gain3/1
  Constant12/1 -> Slider Gain/1, Slider Gain1/1, Slider Gain2/1
  Slider Gain/1 -> Mux2/1
  Slider Gain1/1 -> Mux2/2
  Slider Gain2/1 -> Mux2/3
  Gain3/1 -> PID_FF/1
  Constant6/1 -> Terminator_1/1
  T1/1 -> Gain/1
  Gain/1 -> Mux2/4

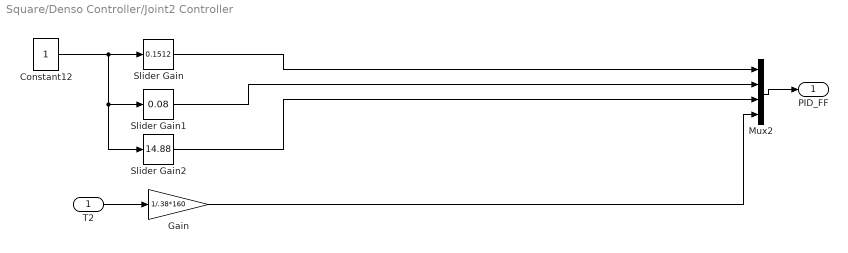
== system Square/Denso Controller/Joint2 Controller ==
  T2 : Inport
  Constant12 : Constant
  Gain : Gain  Gain=1/.38*160
  Mux2 : Mux
  Slider Gain : simulink/Math Operations/Slider Gain  low=0  gain=0.1512  high=1
  Slider Gain1 : simulink/Math Operations/Slider Gain  low=0  gain=0.08  high=0.1
  Slider Gain2 : simulink/Math Operations/Slider Gain  low=0  gain=14.88  high=20
  PID_FF : Outport
  wires:
  Slider Gain2/1 -> Mux2/3
  Slider Gain1/1 -> Mux2/2
  Slider Gain/1 -> Mux2/1
  Constant12/1 -> Slider Gain1/1, Slider Gain2/1, Slider Gain/1
  Mux2/1 -> PID_FF/1
  Gain/1 -> Mux2/4
  T2/1 -> Gain/1

== system Square/Denso Controller/Joint3 Controller ==
  T3 : Inport
  Constant12 : Constant
  Gain : Gain  Gain=1/.38*120
  Mux2 : Mux
  Slider Gain : simulink/Math Operations/Slider Gain  low=0  gain=0.19  high=0.4
  Slider Gain1 : simulink/Math Operations/Slider Gain  low=0  gain=0.3  high=0.5
  Slider Gain2 : simulink/Math Operations/Slider Gain  low=0  gain=10.8  high=18
  PID_FF : Outport
  wires:
  Mux2/1 -> PID_FF/1
  Constant12/1 -> Slider Gain/1, Slider Gain1/1, Slider Gain2/1
  Slider Gain/1 -> Mux2/1
  Slider Gain1/1 -> Mux2/2
  Slider Gain2/1 -> Mux2/3
  T3/1 -> Gain/1
  Gain/1 -> Mux2/4

== system Square/Denso Controller/Joint4 Controller ==
  T4 : Inport
  Constant12 : Constant
  Gain : Gain  Gain=1/.22*100
  Mux2 : Mux
  Slider Gain : simulink/Math Operations/Slider Gain  low=0  gain=0.05  high=0.1
  Slider Gain1 : simulink/Math Operations/Slider Gain  low=0  gain=0.05  high=0.2
  Slider Gain2 : simulink/Math Operations/Slider Gain  low=0  gain=1.4  high=2
  PID_FF : Outport
  wires:
  Gain/1 -> Mux2/4
  Slider Gain2/1 -> Mux2/3
  Slider Gain1/1 -> Mux2/2
  Slider Gain/1 -> Mux2/1
  Constant12/1 -> Slider Gain1/1, Slider Gain2/1, Slider Gain/1
  Mux2/1 -> PID_FF/1
  T4/1 -> Gain/1

== system Square/Denso Controller/Joint5 Controller ==
  T5 : Inport
  Constant12 : Constant
  Gain : Gain  Gain=1/.21*100
  Mux2 : Mux
  Slider Gain : simulink/Math Operations/Slider Gain  low=0  gain=0.182  high=0.2
  Slider Gain1 : simulink/Math Operations/Slider Gain  low=0  gain=0.087  high=0.2
  Slider Gain2 : simulink/Math Operations/Slider Gain  low=0  gain=4.25  high=5
  PID_FF : Outport
  wires:
  Mux2/1 -> PID_FF/1
  Constant12/1 -> Slider Gain/1, Slider Gain1/1, Slider Gain2/1
  Slider Gain/1 -> Mux2/1
  Slider Gain1/1 -> Mux2/2
  Slider Gain2/1 -> Mux2/3
  Gain/1 -> Mux2/4
  T5/1 -> Gain/1

== system Square/Denso Controller/Joint6 Controller ==
  T6 : Inport
  Constant12 : Constant
  Gain : Gain  Gain=1/.21*100
  Mux2 : Mux
  Slider Gain : simulink/Math Operations/Slider Gain  low=0  gain=0.1  high=0.2
  Slider Gain1 : simulink/Math Operations/Slider Gain  low=0  gain=0.1  high=0.1
  Slider Gain2 : simulink/Math Operations/Slider Gain  low=0  gain=3  high=3
  PID_FF : Outport
  wires:
  Slider Gain2/1 -> Mux2/3
  Slider Gain1/1 -> Mux2/2
  Slider Gain/1 -> Mux2/1
  Constant12/1 -> Slider Gain1/1, Slider Gain2/1, Slider Gain/1
  Mux2/1 -> PID_FF/1
  Gain/1 -> Mux2/4
  T6/1 -> Gain/1

== system Square/Denso Controller/Scope Indexing Subsystem The first two inputs are the vectors to be compared. The third input is an index to define the elements in each vector to be compared. ==
  setpoint : Inport
  measured : Inport  Port=2
  index : Inport  Port=3
  Dynamic Router : MATLAB Function  TreatAsAtomicUnit=on
  Dynamic Router1 : MATLAB Function  TreatAsAtomicUnit=on
  Mux2 : Mux  Inputs=2
  Scope : Outport
  Scoped Signal Index : Outport  Port=2
  wires:
  Dynamic Router/1(signal) -> Mux2/1
  Dynamic Router1/1(signal) -> Mux2/2
  index/1 -> Dynamic Router/2(index), Dynamic Router1/2(index), Scoped Signal Index/1
  setpoint/1 -> Dynamic Router/1(array)
  measured/1 -> Dynamic Router1/1(array)
  Mux2/1 -> Scope/1

== system Square/Denso Controller/rising edge latch ==
  rising edge trigger : Inport
  input : Inport  Port=2
  untriggered output : Inport  Port=3
  Latch Input : Subsystem  TreatAsAtomicUnit=on
  Switch : Switch  Threshold=0.5
  output : Outport
  wires:
  untriggered output/1 -> Switch/3
  Switch/1 -> output/1
  Latch Input/1(Latch) -> Switch/1
  Latch Input/2(Executed) -> Switch/2
  input/1 -> Latch Input/1(Input)
  rising edge trigger/1 -> Latch Input/Trigger

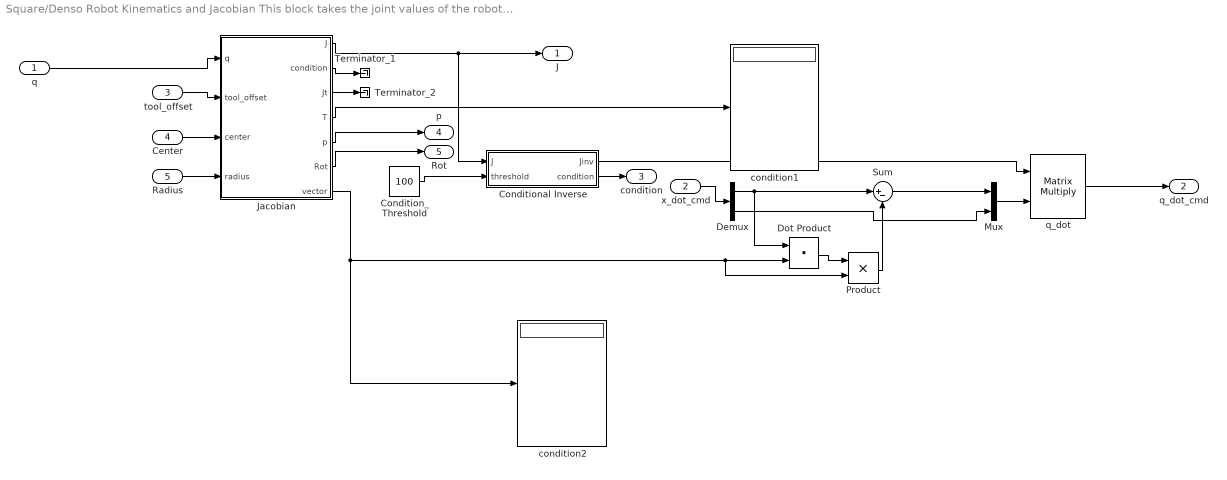
== system Square/Denso Robot Kinematics and Jacobian This block takes the joint values of the robot as the first input and calculates the rotational matrix and position of the robot end-effector in the global frame (first two outputs). It also takes the speed command in the global frame (second input) and converts it to joint speed command (third output)./Jacobian Manipulator ==
  q : Inport
  x_dot_cmd : Inport  Port=2
  tool_offset : Inport  Port=3
  Center : Inport  Port=4
  Radius : Inport  Port=5
  Condition_Threshold : Constant  Value=100
  Conditional Inverse : MATLAB Function  TreatAsAtomicUnit=on
  Demux : Demux  Outputs=[3 3]
  Dot Product : DotProduct  InputSameDT=on  OutDataTypeStr=Inherit: Inherit via internal rule
  Jacobian : MATLAB Function  TreatAsAtomicUnit=on
  Mux : Mux  Inputs=[3 3]
  Product : Product  RndMeth=Zero
  Sum : Sum  Inputs=|+-
  Terminator_1 : Terminator
  Terminator_2 : Terminator
  condition1 : Display
      settings: Decimation=100
  condition2 : Display
      settings: Decimation=100
  q_dot : Product  Multiplication=Matrix(*)  RndMeth=Zero
  J : Outport
  q_dot_cmd : Outport  Port=2
  condition : Outport  Port=3
  p : Outport  Port=4
  Rot : Outport  Port=5
  wires:
  tool_offset/1 -> Jacobian/2(tool_offset)
  Jacobian/1(J) -> J/1, Conditional Inverse/1(J)
  q/1 -> Jacobian/1(q)
  Conditional Inverse/2(condition) -> condition/1
  q_dot/1 -> q_dot_cmd/1
  Condition_Threshold/1 -> Conditional Inverse/2(threshold)
  Jacobian/5(p) -> p/1
  Jacobian/6(Rot) -> Rot/1
  Conditional Inverse/1(Jinv) -> q_dot/1
  Jacobian/2(condition) -> Terminator_1/1
  Jacobian/3(Jt) -> Terminator_2/1
  Jacobian/4(T) -> condition1/1
  Jacobian/7(vector) -> condition2/1, Dot Product/2, Product/2
  Dot Product/1 -> Product/1
  Product/1 -> Sum/2
  x_dot_cmd/1 -> Demux/1
  Demux/1 -> Dot Product/1, Sum/1
  Sum/1 -> Mux/1
  Demux/2 -> Mux/2
  Mux/1 -> q_dot/2
  Center/1 -> Jacobian/3(center)
  Radius/1 -> Jacobian/4(radius)

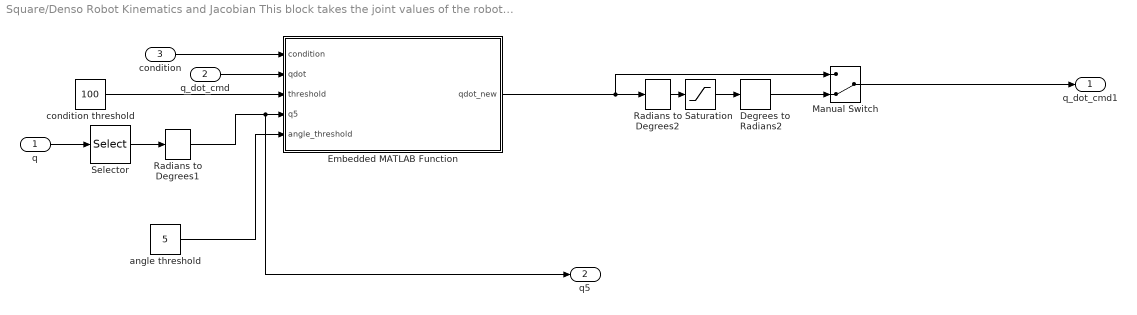
== system Square/Denso Robot Kinematics and Jacobian This block takes the joint values of the robot as the first input and calculates the rotational matrix and position of the robot end-effector in the global frame (first two outputs). It also takes the speed command in the global frame (second input) and converts it to joint speed command (third output)./Singularity Handler ==
  q : Inport
  q_dot_cmd : Inport  Port=2
  condition : Inport  Port=3
  Degrees to Radians2 : simulink_extras/Transformations/Degrees to Radians
  Embedded MATLAB Function : MATLAB Function  TreatAsAtomicUnit=on
  Manual Switch : ManualSwitch  CurrentSetting=0
  Radians to Degrees1 : simulink_extras/Transformations/Radians to Degrees
  Radians to Degrees2 : simulink_extras/Transformations/Radians to Degrees
  Saturation : Saturate  UpperLimit=180  LowerLimit=-180
  Selector : Selector  InputPortWidth=6  IndexOptions=Index vector (dialog)  Indices=5  OutputSizes=1
  angle threshold : Constant  Value=5
  condition threshold : Constant  Value=100
  q_dot_cmd1 : Outport
  q5 : Outport  Port=2
  wires:
  Saturation/1 -> Degrees to Radians2/1
  Radians to Degrees2/1 -> Saturation/1
  Degrees to Radians2/1 -> Manual Switch/2
  Manual Switch/1 -> q_dot_cmd1/1
  condition/1 -> Embedded MATLAB Function/1(condition)
  q_dot_cmd/1 -> Embedded MATLAB Function/2(qdot)
  condition threshold/1 -> Embedded MATLAB Function/3(threshold)
  Embedded MATLAB Function/1(qdot_new) -> Radians to Degrees2/1, Manual Switch/1
  q/1 -> Selector/1
  Selector/1 -> Radians to Degrees1/1
  angle threshold/1 -> Embedded MATLAB Function/5(angle_threshold)
  Radians to Degrees1/1 -> Embedded MATLAB Function/4(q5), q5/1

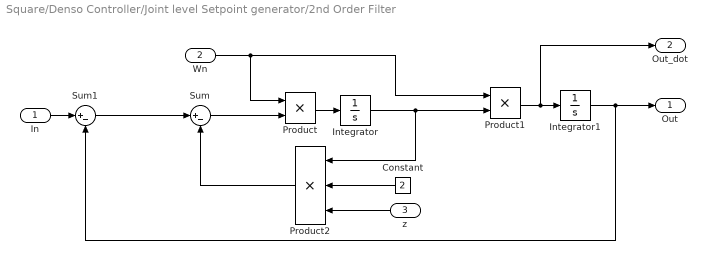
== system Square/Denso Controller/Joint level Setpoint generator/2nd Order Filter ==
  In : Inport
  Wn : Inport  Port=2
  z : Inport  Port=3
  Constant : Constant  Value=2
  Integrator : Integrator
  Integrator1 : Integrator
  Product : Product  RndMeth=Zero
  Product1 : Product  RndMeth=Zero
  Product2 : Product  Inputs=3  RndMeth=Zero
  Sum : Sum  Inputs=|+-
  Sum1 : Sum  Inputs=|+-
  Out : Outport
  Out_dot : Outport  Port=2
  wires:
  Product/1 -> Integrator/1
  Sum/1 -> Product/2
  Wn/1 -> Product/1, Product1/1
  Product1/1 -> Integrator1/1, Out_dot/1
  Integrator/1 -> Product1/2, Product2/1
  Integrator1/1 -> Sum1/2, Out/1
  Sum1/1 -> Sum/1
  In/1 -> Sum1/1
  Product2/1 -> Sum/2
  z/1 -> Product2/3
  Constant/1 -> Product2/2

== system Square/Denso Controller/Joint level Setpoint generator/Linear Trajectory Maker. ==
  Desired : Inport
  Initial : Inport  Port=2
  Speed : Inport  Port=3
  Enable : EnablePort  StatesWhenEnabling=reset
  Linear Trajectory : Subsystem  Priority=1  AncestorBlock=quanser_tunable_functions/Linear Trajectory
  Command : Outport  OutputWhenDisabled=reset  InitialOutput=zeros (1,6)
  wires:
  Desired/1 -> Linear Trajectory/1(desired)
  Initial/1 -> Linear Trajectory/2(initial)
  Speed/1 -> Linear Trajectory/3(speed)
  Linear Trajectory/1(trajectory) -> Command/1

== system Square/Denso Controller/rising edge latch/Latch Input ==
  Input : Inport
  Trigger : TriggerPort
  Constant : Constant
  Latch : Outport
  Executed : Outport  Port=2
  wires:
  Constant/1 -> Executed/1
  Input/1 -> Latch/1

== system Square/Denso Controller/Joint level Setpoint generator/Linear Trajectory Maker./Linear Trajectory ==
  desired : Inport
  initial : Inport  Port=2
  speed : Inport  Port=3
  Constant2 : Constant  Value=qc_get_step_size
  Embedded MATLAB Function : MATLAB Function  TreatAsAtomicUnit=on
  Unit Delay External IC : simulink/Additional Math & Discrete/Additional Discrete/Unit Delay External IC  tsamp=-1
  trajectory : Outport
  wires:
  initial/1 -> Unit Delay External IC/2
  speed/1 -> Embedded MATLAB Function/3(speed)
  desired/1 -> Embedded MATLAB Function/1(final)
  Constant2/1 -> Embedded MATLAB Function/4(sample_time)
  Embedded MATLAB Function/1(inter) -> trajectory/1, Unit Delay External IC/1
  Unit Delay External IC/1 -> Embedded MATLAB Function/2(current)

== matlab function Square/Denso Controller/Joint level Setpoint generator/Linear Trajectory Maker./Linear Trajectory/Embedded MATLAB Function ==
  data: final input; inter output; current input; speed input; sample_time input
function inter = linear_interpolator( final, current, speed, sample_time)

step = speed*sample_time;
inter = current + sign(final-current).*step;


for i = 1:length(final)
    if ( abs (final(i)-current(i)) < step(i))
        inter(i) = final(i);
    end
end
end

== matlab function Square/Denso Robot Kinematics and Jacobian This block takes the joint values of the robot as the first input and calculates the rotational matrix and position of the robot end-effector in the global frame (first two outputs). It also takes the speed command in the global frame (second input) and converts it to joint speed command (third output)./Jacobian Manipulator/Jacobian ==
  data: q input; J output; tool_offset input; condition output; Jt output; T output; p output; Rot output; center input; radius input; vector output
function [J, condition, Jt,  T, p,Rot,vector] = Denso_Kinematics(q, tool_offset,center,radius)

l1z = 125*1e-3;
l1x = 0;
l2 = 210*1e-3;
l3z = 88*1e-3;
l3x = 75*1e-3;
l4 = 122*1e-3;
l5 = 70*1e-3;

A1 = DH (q(1), l1z, l1x, pi/2);
A2 = DH (q(2) + pi/2, 0, l2, 0);
A3 = DH (q(3) - pi/2, 0, -l3x, -pi/2);
A4 = DH (q(4), l3z+l4, 0, pi/2);
A5 = DH (q(5), 0, 0, -pi/2);
A6 = DH (q(6), l5, 0, 0);

z0 = [0 0 1]';
p0 = [0 0 0]';
z1 = A1(1:3,3);
p1 = A1(1:3,4);
T2 = A1*A2;
z2 = T2(1:3,3);
p2 = T2(1:3,4);
T3 = A1*A2*A3;
z3 = T3(1:3,3);
p3 = T3(1:3,4);
T4 = A1*A2*A3*A4;
z4 = T4(1:3,3);
p4 = T4(1:3,4);
T5 = A1*A2*A3*A4*A5;
z5 = T5(1:3,3);
p5 = T5(1:3,4);
T6 = A1*A2*A3*A4*A5*A6;
z6 = T6(1:3,3);
p6 = T6(1:3,4);
T_tool = T6 * tool_offset;
p = T_tool(1:3);

T = p5;%T2(1:3,1);
Rot = T6(1:3,1:3);

J = [cross(z0,(p-p0)) cross(z1,(p-p1)) cross(z2,(p-p2)) cross(z3,(p-p3)) cross(z4,(p-p4)) cross(z5,(p-p5))
    z0 z1 z2 z3 z4 z5];

Jt = J';

%J_inv = inv(J);
condition = cond (J);

if sqrt((p5(1)-center(1))^2 + (p5(2)-center(2))^2 +(p5(3)-center(3))^2)>radius
    vector = (p5-center)/norm(p5-center);
else 
    vector = [0; 0; 0];
end

end

function A = DH(theta_z, d_z, a_x, alpha_x)

A_R_z = [cos(theta_z) -sin(theta_z) 0 0;
         sin(theta_z) cos(theta_z) 0 0;
         0 0 1 0;
         0 0 0 1];

A_T_z = [1 0 0 0;
         0 1 0 0;
         0 0 1 d_z;
         0 0 0 1];

A_T_x = [1 0 0 a_x;
         0 1 0 0;
         0 0 1 0;
         0 0 0 1];

A_R_x = [1 0 0 0;
         0 cos(alpha_x) -sin(alpha_x)  0;
         0 sin(alpha_x) cos(alpha_x) 0;
         0 0 0 1];

A = A_R_z*A_T_z*A_T_x*A_R_x;
end

== matlab function Square/Denso Controller/Scope Indexing Subsystem The first two inputs are the vectors to be compared. The third input is an index to define the elements in each vector to be compared./Dynamic Router1 ==
  data: array input; signal output; index input
function signal = Route(array,index)
signal = array(index);

== matlab function Square/Denso Robot Kinematics and Jacobian This block takes the joint values of the robot as the first input and calculates the rotational matrix and position of the robot end-effector in the global frame (first two outputs). It also takes the speed command in the global frame (second input) and converts it to joint speed command (third output)./Singularity Handler/Embedded MATLAB Function ==
  data: condition input; qdot_new output size=6; qdot input size=6; threshold input; q5 input; angle_threshold input
function qdot_new = wrist_handler(condition, qdot, threshold, q5, angle_threshold)
qdot_new = qdot;
if ( (condition > threshold) && (abs(q5) < angle_threshold) ) 
% if (condition > threshold) 
    qdot_new(1) = qdot(1);
    qdot_new(2) = qdot(2);
    qdot_new(3) = qdot(3);
    qdot_new(4) = 0;
    qdot_new(5) = qdot(5);
    qdot_new(6) = qdot(4)+qdot(6);
end
end

== matlab function Square/Denso Robot Kinematics and Jacobian This block takes the joint values of the robot as the first input and calculates the rotational matrix and position of the robot end-effector in the global frame (first two outputs). It also takes the speed command in the global frame (second input) and converts it to joint speed command (third output)./Jacobian Manipulator/Conditional Inverse ==
  data: J input; Jinv output; condition output; threshold input
function [Jinv, condition] = myinv(J, threshold)
% tolerance = MAX(size(J)) * NORM(J) * EPS(class(J));
condition = cond(J);
if (condition > threshold)
    Jinv = pinv(J);
else
    Jinv = inv(J);
end
end

== matlab function Square/Denso Robot Kinematics and Jacobian This block takes the joint values of the robot as the first input and calculates the rotational matrix and position of the robot end-effector in the global frame (first two outputs). It also takes the speed command in the global frame (second input) and converts it to joint speed command (third output)./Embedded MATLAB Function ==
  data: r input; rx output; ry output; rz output
function [rx,ry,rz] = Fixed_Frame(r)
rz = atan2(r(2,1) ,r(1,1));
ry = atan2 (-r(3,1), sqrt(r(3,2)^2 + r(3,3)^2));
rx = atan2(r(3,2), r(3,3));
end

== matlab function Square/Denso Controller/Scope Indexing Subsystem The first two inputs are the vectors to be compared. The third input is an index to define the elements in each vector to be compared./Dynamic Router ==
  data: array input; signal output; index input
function signal = Route(array,index)
signal = array(index);
